simulink model "quadrotor_from_scratch"  (R2026a)
settings: Solver=ode45  MaxStep=0.01  RelTol=1e-6
settings Model: Creator=ASUS  LastModifiedBy=ASUS

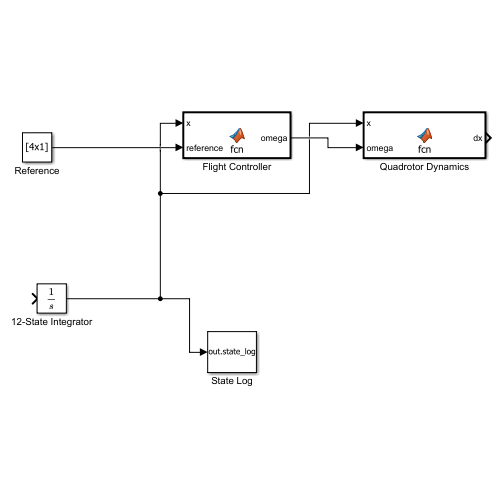
[thumbnail: Simulink's stored preview of the top-level diagram]
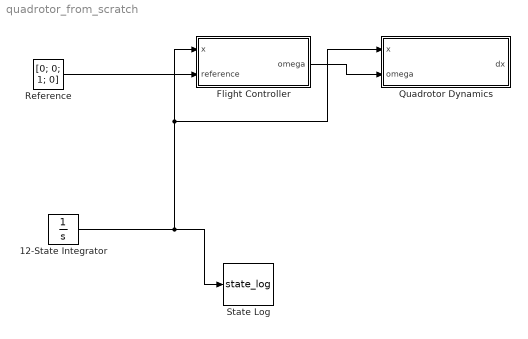
== system quadrotor_from_scratch ==
  12-State Integrator : Integrator  InitialCondition=zeros(12,1)
  Flight Controller : MATLAB Function  TreatAsAtomicUnit=on
  Quadrotor Dynamics : MATLAB Function  TreatAsAtomicUnit=on
  Reference : Constant  Value=[0; 0; 1; 0]
  State Log : ToWorkspace  VariableName=state_log  SaveFormat=Timeseries  SampleTime=-1
      settings: Save2DSignal=2-D array (concatenate along first dimension)
  wires:
  Reference/1 -> Flight Controller/2(reference)
  Flight Controller/1(omega) -> Quadrotor Dynamics/2(omega)
  12-State Integrator/1 -> State Log/1, Flight Controller/1(x), Quadrotor Dynamics/1(x)

== matlab function quadrotor_from_scratch/Flight Controller ==
  data: x input; omega output; reference input
function omega = fcn(x, reference)
%#codegen
omega = flightController(x, reference);
end

== matlab function quadrotor_from_scratch/Quadrotor Dynamics ==
  data: x input; dx output; omega input
function dx = fcn(x, omega)
%#codegen
dx = quadDynamics(x, omega);
end
